simulink model "multilevel_inverter"  (Simulink 8.7)
settings: Solver=VariableStepAuto  StartTime=0.0  StopTime=0.2  RelTol=1e-3
libraries: powerlib x13
settings Model: Creator=Rohith  LastModifiedBy=Rohith
settings DataIOCC: LimitDataPoints=off  SaveFormat=Dataset
settings DebuggingCC: UnderspecifiedInitializationDetection=Simplified  MergeDetectMultiDrivingBlocksExec=error
settings HardwareCC: ProdBitPerPointer=64  ProdLargestAtomicFloat=Float  ProdIntDivRoundTo=Zero  ProdEndianess=LittleEndian  ProdWordSize=64  ProdHWDeviceType=Intel->x86-64 (Windows64)
settings ModelReferenceCC: PropagateSignalLabelsOutOfModel=on
settings ConfigComp: CovModelRefEnable=off

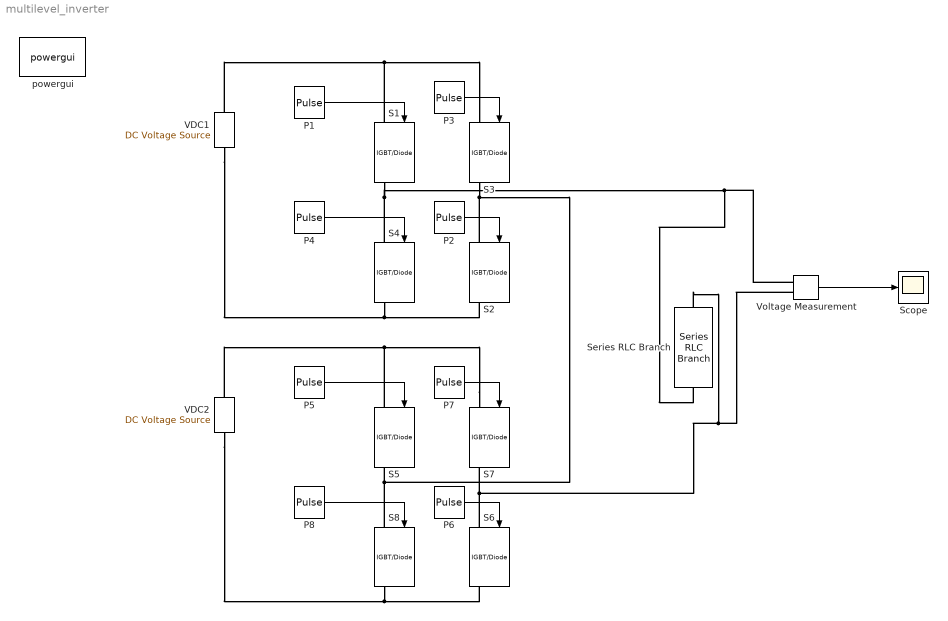
== system multilevel_inverter ==
  "  S3" : powerlib/Power Electronics/IGBT//Diode  Ron=1e-3  Rs=1e5  Cs=inf  Measurements=on
  "  S7" : powerlib/Power Electronics/IGBT//Diode  Ron=1e-3  Rs=1e5  Cs=inf  Measurements=on
  P1 : DiscretePulseGenerator  PulseType=Time based  Period=0.02  PulseWidth=30  PhaseDelay=0.002
  P2 : DiscretePulseGenerator  PulseType=Time based  Period=0.02  PulseWidth=30  PhaseDelay=0.002
  P3 : DiscretePulseGenerator  PulseType=Time based  Period=0.02  PulseWidth=10  PhaseDelay=0.014
  P4 : DiscretePulseGenerator  PulseType=Time based  Period=0.02  PulseWidth=30  PhaseDelay=0.012
  P5 : DiscretePulseGenerator  PulseType=Time based  Period=0.02  PulseWidth=10  PhaseDelay=0.004
  P6 : DiscretePulseGenerator  PulseType=Time based  Period=0.02  PulseWidth=30  PhaseDelay=0.002
  P7 : DiscretePulseGenerator  PulseType=Time based  Period=10  PulseWidth=5  PhaseDelay=0.012
  P8 : DiscretePulseGenerator  PulseType=Time based  Period=0.02  PulseWidth=30  PhaseDelay=0.012
  S{1..2,5..6,8} (5 alike) : powerlib/Power Electronics/IGBT//Diode  Ron=1e-3  Rs=1e5  Cs=inf  Measurements=on
  "S4 " : powerlib/Power Electronics/IGBT//Diode  Ron=1e-3  Rs=1e5  Cs=inf  Measurements=on
  Scope : Scope
  Series RLC Branch : powerlib/Elements/Series RLC Branch  LConnTagsString=__new0  RConnTagsString=__new0  BranchType=R  Resistance=10  Inductance=1e-3  SetiL0=off  InitialCurrent=0  Capacitance=1e-6  Setx0=off  InitialVoltage=0  Measurements=None
  VDC1 : powerlib/Electrical Sources/DC Voltage Source  Amplitude=100  Measurements=None
  VDC2 : powerlib/Electrical Sources/DC Voltage Source  Amplitude=100  Measurements=None
  Voltage Measurement : powerlib/Measurements/Voltage Measurement  PhasorSimulation=off  OutputType=Complex  PSBequivalent=0
  powergui : powerlib/powergui  Priority=1  SimulationMode=Continuous  SolverType=Tustin/Backward Euler (TBE)  SampleTime=50e-6  frequency=60  SPID=off  DisableSnubberDevices=off  DisableRonSwitches=off  DisableVfSwitches=off  SwTol=0  DisplayEquations=off  Interpol=off  ExternalGateDelay=off  methode=off  Ts=10  FunctionMessages=off  echomessages=off  HookPort=off  EnableUseOfTLC=off  x0status=blocks  frequencyindice=0  Pbase=100e6  ErrMax=1e-4  Iterations=50  UnitsV=kV  UnitsW=MW  buscounter=0  RestoreLinks=warning  ResistiveCurrentMeasurement=off  Frange=[0:2:500]  Ylog=off  Xlog=on  ShowGrid=off  save=off  variable=ZData  structure=0  ZoomFFT=off  StartTime=0.0  cycles=1  DisplayStyle=1  fundamental=60  FreqAxis=off  MaxFrequency=1000  frequencyindicesteady=1  RmsSteady=1  display=off
  wires:
  P1/1 -> S1/1
  P4/1 -> "S4 "/1
  P3/1 -> "  S3"/1
  P2/1 -> S2/1
  P5/1 -> S5/1
  P8/1 -> S8/1
  P7/1 -> "  S7"/1
  P6/1 -> S6/1
  Voltage Measurement/1 -> Scope/1
  connections:
  VDC1/RConn1 -- S1/LConn1 -- "  S3"/LConn1
  VDC1/LConn1 -- "S4 "/RConn1 -- S2/RConn1
  "  S7"/LConn1 -- S5/LConn1 -- VDC2/RConn1
  VDC2/LConn1 -- S8/RConn1 -- S6/RConn1
  S8/LConn1 -- S2/LConn1 -- "  S3"/RConn1 -- S5/RConn1
  S6/LConn1 -- Voltage Measurement/LConn2 -- Series RLC Branch/RConn1 -- "  S7"/RConn1
  S1/RConn1 -- Voltage Measurement/LConn1 -- Series RLC Branch/LConn1 -- "S4 "/LConn1
